simulink model "spaceshipWSINOUT"  (Simulink 6.1)
settings: Solver=ode45  StartTime=0.0  StopTime=10.0  RelTol=1e-3
settings Model: LastModifiedBy=okawa
settings DebuggingCC: SolverPrmCheckMsg=warning

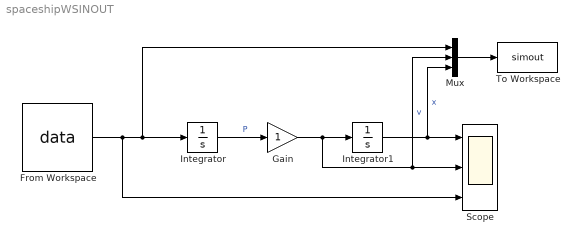
== system spaceshipWSINOUT ==
  From Workspace : FromWorkspace  VariableName=data  SampleTime=0.01
  Gain : Gain
  Integrator : Integrator
  Integrator1 : Integrator
  Mux : Mux  Inputs=3
  Scope : Scope  NumInputPorts=3
      settings: YMin=-5~-5~-5  YMax=5~5~5
  To Workspace : ToWorkspace  VariableName=simout  SampleTime=-1  SaveFormat=Array
  wires:
  Integrator1/1 -> Scope/1, Mux/3  "x"
  Integrator/1 -> Gain/1  "P"
  Gain/1 -> Integrator1/1, Scope/2, Mux/2  "v"
  Mux/1 -> To Workspace/1
  From Workspace/1 -> Integrator/1, Mux/1, Scope/3
